simulink model "z_pmsm_basic_input"  (R2022a)
settings: Solver=VariableStepAuto  StartTime=0.0  StopTime=10.0  RelTol=1e-3
libraries: mcbpositiondecoderlib x1, autolibpmsmexterior x1
settings Model: Creator=yusuf.ogut  LastModifiedBy=yusuf.ogut

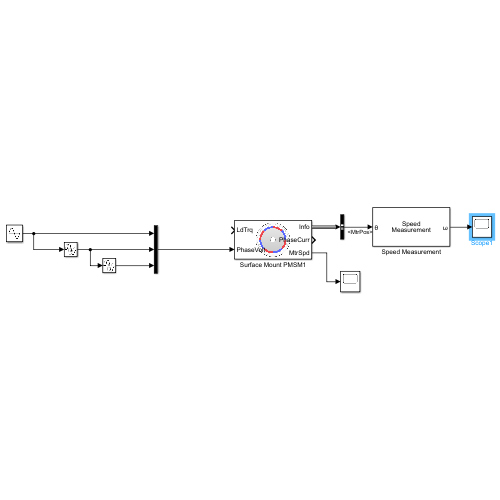
[thumbnail: Simulink's stored preview of the top-level diagram]
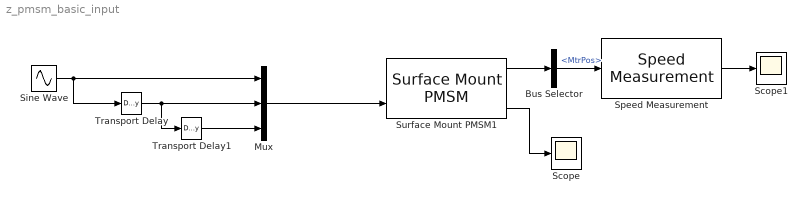
== system z_pmsm_basic_input ==
  Bus Selector : BusSelector  OutputSignals=MtrPos
  Mux : Mux  Inputs=3
  Scope : Scope
  Scope1 : Scope
  Sine Wave : Sin  Amplitude=28  SampleTime=0
  Speed Measurement : mcbpositiondecoderlib/Speed Measurement  PositionUnit=Radians  PositionScalingDatatype=uint32  SpeedCalculationMode=Maximum application speed  SampleTimeAsync=100e-6  MaximumApplicationSpeed=1000  SpeedResolution=5e-6  DelayLength=299  MaximumMeasurableSpeed=1000  MeasurableSpeedResolution=4.6566e-07  SpeedUnit=RPM  PerUnitSpeed=1000  SpeedDataType=single
      settings: SourceProductBaseCode=MT
  Surface Mount PMSM1 : autolibpmsmexterior/Surface Mount PMSM  port_config=Torque  sim_type=Continuous  Ts=0.001  P=2  Rs=15e-03  Ldq_=13.5e-06  KConstText=Torque constant (Kt):  lambda_pm=0.2205  Ke=25  Kt=0.04  mechanical=[2.584e-04, 2.5e-04, 0]  idq0=[0 0]  theta_init=0  omega_init=0  KConst=0.04  lambda_pm_calc=0.013333  RefBlkName='autolibpmsmexterior/Surface Mount PMSM'  aMode=5  Ldq="[0.0017      0.0017]"
      settings: SourceProductBaseCode=PW,DR,MT,VE
  Transport Delay : TransportDelay
  Transport Delay1 : TransportDelay
  wires:
  Sine Wave/1 -> Transport Delay/1, Mux/1
  Transport Delay/1 -> Transport Delay1/1, Mux/2
  Transport Delay1/1 -> Mux/3
  Mux/1 -> Surface Mount PMSM1/2
  Surface Mount PMSM1/3 -> Scope/1
  Surface Mount PMSM1/1 -> Bus Selector/1
  Bus Selector/1 -> Speed Measurement/1  "<MtrPos>"
  Speed Measurement/1 -> Scope1/1
